simulink model "cse2"  (Simulink 7.7)
settings: Solver=ode45  StartTime=0.0  StopTime=10.0  RelTol=1e-3
values from neighbouring files (symbols this model uses):
  k_d = 0.02    [case2.m]
  k_i = 0.0003    [case2.m]
  k_p = .04    (= 0.04)    [case2.m]
  N = .1    (= 0.1)    [case2.m]
settings Model: Creator=Edward  LastModifiedBy=Edward

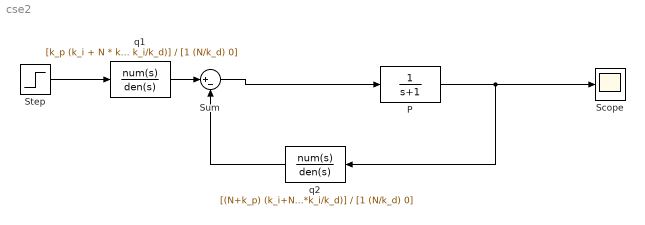
== system cse2 ==
  P : TransferFcn  Denominator=[1 1]
  Scope : Scope
  Step : Step  SampleTime=0
  Sum : Sum  Inputs=|+-
  q1 : TransferFcn  Numerator=[k_p (k_i + N * k_p/k_d) + (N * k_i/k_d)]  Denominator=[1 (N/k_d) 0]
  q2 : TransferFcn  Numerator=[(N+k_p) (k_i+N*k_p/k_d) (N*k_i/k_d)]  Denominator=[1 (N/k_d) 0]
  wires:
  Sum/1 -> P/1
  q1/1 -> Sum/1
  q2/1 -> Sum/2
  P/1 -> Scope/1, q2/1
  Step/1 -> q1/1
